simulink model "Set_Speed_Harness"  (R2022b)
settings: configuration reference "CommonModelConfiguration" (kept outside this file)
(part 3 of 3)

== stateflow chart Set_Speed_Harness/Test Sequence ==
  state Initialize_
    INT_SWSInputData.Button = E_SWSEvent_Idle;
    INT_SWSInputData.Event = E_SWSEvent_Idle;
    GET_VehSpdIndcdVal = double(0);
    GET_SpdUnit = VehSpdIndcdUnit.VehSpdIndcdUnit_UkwnUnit;
    PA_DSF_Speed_Limiter_Status = E_CommonStatus.NotPresent;
    PA_DSF_Speed_Limiter_Value = E_DSF_Value.DSF_Off;
    PA_DSF_Cruise_Control_Status = E_CommonStatus.NotPresent;
    PA_DSF_Cruise_Control_Value = E_DSF_Value.DSF_Off;
    PA_DSF_Adaptive_Cruise_Control_Status = E_CommonStatus.NotPresent;
    PA_DSF_Adaptive_Cruise_Control_Value = E_DSF_Value.DSF_Off;
    GET_SetSpdSelnForAutDrv = SetSpdSelnForAutDrv1.SetSpdSelnForAutDrv1_KeepSetSpdValPrsnt;
    GET_SpdLimUnit = SpdUnit1.SpdUnit1_KiloMtrPerHr;
    INT_CC_Event = E_DSF_Event.NoReq;
    INT_SL_Event = E_DSF_Event.NoReq;
    INT_ACC_Event = E_DSF_Event.NoReq;
    GET_CrsCtrlOvrdn = OnOff1.OnOff1_Off;
    PA_DSF_Speed_Limit_Adaptation_Value = E_DSF_Value.DSF_Off;
    PA_DSF_Speed_Limit_Adaptation_Data = double(0);
    PA_DSF_SL_Warning_Value = E_OffOn.Off;
    GET_AdjSpdLimnSts = AdjSpdLimnSts2.AdjSpdLimnSts2_Off;
    GET_UsrSeldDrvrSpprtFct = DrvrSpprtFct.DrvrSpprtFct_NoReq;
    GET_HmiAutnmsSts = HmiAutnmsSts1.HmiAutnmsSts1_Ukwn;
    GET_AccSts = AccSts1.AccSts1_Off;
    PA_VS_ReducedMaxSpeed_Status = E_CommonStatus.NotPresent;
    GET_KeyRstrictdActvSpeedLimit = double(0);
    PA_SpeedControlFunction_Status = E_CommonStatus.NotPresent;
    PA_SpeedControlFunction_Data = double(0);
    PA_SpeedControlFunction_Value = E_OffOn.Off;
  state TC1_SS_NormalOperation_ACC_Available
    state TC1_NormalOperation_1
      GET_UsrSeldDrvrSpprtFct = DrvrSpprtFct.DrvrSpprtFct_ACC;
      PA_DSF_Adaptive_Cruise_Control_Status = E_CommonStatus.Available;
      GET_HmiAutnmsSts = HmiAutnmsSts1.HmiAutnmsSts1_On;
      PA_VS_ReducedMaxSpeed_Status = E_CommonStatus.NotPresent;  % Many combination possible
      GET_SpdUnit = VehSpdIndcdUnit.VehSpdIndcdUnit_Kmph;
      PA_DSF_Adaptive_Cruise_Control_Value = E_DSF_Value.DSF_Active;
      INT_ACC_Event = E_DSF_Event.NoReq;
      INT_SWSInputData.Event = E_SWSEvent_Idle;
      GET_AccSts = AccSts1.AccSts1_Actv; % Activation of ACC thru Public Attribute
      PA_DSF_Speed_Limit_Adaptation_Value = E_DSF_Value.DSF_Off
    state Set_current_speed
      PA_DSF_Adaptive_Cruise_Control_Status = E_CommonStatus.Available;
      GET_CrsCtrlOvrdn = OnOff1.OnOff1_On;
      INT_SWSInputData.Button = E_SWSButton_BtnL5Req;
      INT_SWSInputData.Event = E_SWSEvent_Push;
      GET_VehSpdIndcdVal = double(70);
    state SWS_event_to_idle
      INT_SWSInputData.Event = E_SWSEvent_Idle;
    state Inputs_for_SPEED_TAP
      INT_SWSInputData.Event= E_SWSEvent_Release;
      INT_SWSInputData.Button= E_SWSButton_BtnL5Req;
    state SWS_event_to_idle1
      INT_SWSInputData.Event = E_SWSEvent_Idle;
    state Inputs_for_SPEED_RAMP
      INT_SWSInputData.Event= E_SWSEvent_HoldShort;
      INT_SWSInputData.Button= E_SWSButton_BtnL4Req;
    state Button_release
      INT_SWSInputData.Event= E_SWSEvent_Release;
    (default) -> TC1_NormalOperation_1
    TC1_NormalOperation_1 -> Set_current_speed : [
        | after(1,sec)
        | ]
    Set_current_speed -> SWS_event_to_idle : [
        | after(1,sec)
        | ]
    SWS_event_to_idle -> Inputs_for_SPEED_TAP : [
        | after(2,sec)
        | ]
    Inputs_for_SPEED_TAP -> SWS_event_to_idle1 : [
        | after(5,sec)
        | ]
    SWS_event_to_idle1 -> Inputs_for_SPEED_RAMP : [
        | after(2,sec)
        | ]
    Inputs_for_SPEED_RAMP -> Button_release : [
        | after(2,sec)
        | ]
  state TC1_SS_NormalOperation_CC_Available
    state TC1_CC_NormalOeration_1
      PA_DSF_Adaptive_Cruise_Control_Value = E_DSF_Value.DSF_Off;
      PA_DSF_Cruise_Control_Value = E_DSF_Value.DSF_Active;
    (default) -> TC1_CC_NormalOeration_1
  (default) -> Initialize_
  Initialize_ -> TC1_SS_NormalOperation_ACC_Available : [
      | after(2, sec)
      | ]
  data: INT_SWSInputData output Bus: SWSInputData; GET_VehSpdIndcdVal output; GET_SpdUnit output; PA_DSF_Speed_Limiter_Status output; PA_DSF_Speed_Limiter_Value output; PA_DSF_Cruise_Control_Status output; PA_DSF_Cruise_Control_Value output; PA_DSF_Adaptive_Cruise_Control_Status output; PA_DSF_Adaptive_Cruise_Control_Value output; GET_SetSpdSelnForAutDrv output; GET_SpdLimUnit output; INT_CC_Event output; INT_SL_Event output; INT_ACC_Event output; GET_CrsCtrlOvrdn output; PA_DSF_Speed_Limit_Adaptation_Value output; PA_DSF_Speed_Limit_Adaptation_Data output; PA_DSF_SL_Warning_Value output; GET_AdjSpdLimnSts output; GET_UsrSeldDrvrSpprtFct output; GET_HmiAutnmsSts output; GET_AccSts output; PA_VS_ReducedMaxSpeed_Status output; GET_KeyRstrictdActvSpeedLimit output; PA_SpeedControlFunction_Status output; PA_SpeedControlFunction_Data output; PA_SpeedControlFunction_Value output; E_SWSEvent_Idle constant double =0; E_SWSEvent_Push constant double =1; E_SWSEvent_Release constant double =2; E_SWSEvent_HoldShort constant double =3; E_SWSEvent_HoldLong constant double =4; E_SWSEvent_ButtonStuck constant double =5; E_SWSEvent_Deactivation constant double =6; E_SWSButton_BtnL1Req constant double =1; E_SWSButton_BtnL2Req constant double =2; E_SWSButton_BtnL3Req constant double =3; E_SWSButton_BtnL4Req constant double =4; E_SWSButton_BtnL5Req constant double =5; E_SWSButton_BtnL6Req constant double =6; E_SWSButton_BtnL7Req constant double =7
